simulink model "one"  (R2021a)
settings: Solver=ode45  StartTime=0.0  StopTime=50.0  MaxStep=0.05  RelTol=1e-3
libraries: pid_lib x1
settings Model: Creator=jeffr  LastModifiedBy=jeffr

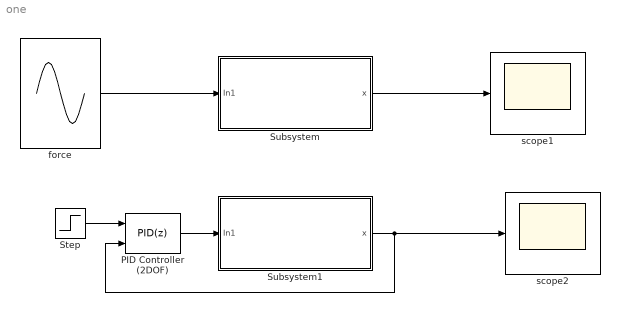
== system one ==
  PID Controller (2DOF) : pid_lib/PID Controller (2DOF)  Controller=PID  Form=Parallel  TimeDomain=Discrete-time  UseExternalTs=off  SampleTime=0.01  IntegratorMethod=Forward Euler  FilterMethod=Forward Euler  ControllerParametersSource=internal  P=1  I=1  D=0  UseFilter=on  N=100  b=1  c=1  TunerSelectOption=Transfer Function Based (PID Tuner App)  InitialConditionSource=internal  InitialConditionForIntegrator=0  InitialConditionForFilter=0  DifferentiatorICPrevScaledInput=0  ExternalReset=none  TrackingMode=off  Kt=1  LimitOutput=off  SatLimitsSource=internal  UpperSaturationLimit=inf  LowerSaturationLimit=-inf  LinearizeAsGain=on  AntiWindupMode=none  Kb=1  POutMin=[]  POutMax=[]  IOutMin=[]  IOutMax=[]  DOutMin=[]  DOutMax=[]  NOutMin=[]  NOutMax=[]  bOutMin=[]  bOutMax=[]  cOutMin=[]  cOutMax=[]  SumOutMin=[]  SumOutMax=[]  SaturationOutMin=[]  SaturationOutMax=[]  PParamMin=[]  PParamMax=[]  IParamMin=[]  IParamMax=[]  DParamMin=[]  DParamMax=[]  NParamMin=[]  NParamMax=[]  bParamMin=[]  bParamMax=[]  cParamMin=[]  cParamMax=[]  KbParamMin=[]  KbParamMax=[]  KtParamMin=[]  KtParamMax=[]  KbOutMin=[]  KbOutMax=[]  KtOutMin=[]  KtOutMax=[]  IntegratorOutMin=[]  IntegratorOutMax=[]  FilterOutMin=[]  FilterOutMax=[]  SumI1OutMin=[]  SumI1OutMax=[]  SumI2OutMin=[]  SumI2OutMax=[]  SumI3OutMin=[]  SumI3OutMax=[]  SumI4OutMin=[]  SumI4OutMax=[]  SumDOutMin=[]  SumDOutMax=[]  Sum1OutMin=[]  Sum1OutMax=[]  Sum2OutMin=[]  Sum2OutMax=[]  Sum3OutMin=[]  Sum3OutMax=[]  DifferentiatorOutMin=[]  DifferentiatorOutMax=[]  FilterDiffOutCoefMin=[]  FilterDiffOutCoefMax=[]  ReciprocalOutMin=[]  ReciprocalOutMax=[]  SumDenOutMin=[]  SumDenOutMax=[]  SumNumOutMin=[]  SumNumOutMax=[]  DivideOutMin=[]  DivideOutMax=[]  UdiffTsProdOutMin=[]  UdiffTsProdOutMax=[]  NTsProdOutMin=[]  NTsProdOutMax=[]  UintegralTsProdOutMin=[]  UintegralTsProdOutMax=[]  UngainTsProdOutMin=[]  UngainTsProdOutMax=[]  IntegratorContinuousStateAttributes=''  IntegratorStateMustResolveToSignalObject=off  IntegratorRTWStateStorageClass=Auto  FilterContinuousStateAttributes=''  FilterStateMustResolveToSignalObject=off  FilterRTWStateStorageClass=Auto  ParallelPVariant=InternalParameters  IdealPVariant=Disabled  IVariant=InternalParameters  DVariant=InternalParameters  bVariant=InternalParameters  cVariant=InternalParameters  IntegratorVariant=Discrete  SatVariant=Disabled  AWVariant=Passthrough  PCopyVariant=Disabled  TRVariant=Disabled  FdbkBlocksVariant=Forward  IdealPFdbkVariant=Disabled  SatFdbkVariant=Disabled  DerivativeFilterVariant=ForwardEulerFilter  NVariant=InternalParameters  NCopyVariant=Disabled  FilterICVariant=InternalICsFilter  IntegratorICVariant=InternalICs  ExternalResetVariant=Disabled  TRSumVariant=Passthrough  SumFdbkVariant=Disabled  SumVariant=Sum_PID  TsampFilterVariant=InternalTs  TsampNgainVariant=Passthrough  TsampIntegralVariant=Passthrough  ExternalSaturationOutDataTypeStr=Inherit: Same as second input
      settings: SourceProductBaseCode=SL
  Step : Step  SampleTime=0
  Subsystem : Subsystem  mask{m=1, k=0.2, b=0.1}
      mask prompts: m "mass"; k "spring"; b "damper"
      mask Display: disp('my subsystem')
  Subsystem1 : Subsystem  mask{m=1, k=0.2, b=0.1}
      mask prompts: m "mass"; k "spring"; b "damper"
      mask Display: disp('my subsystem')
  force : Sin  Amplitude=2  SampleTime=0
  scope1 : Scope
  scope2 : Scope
  wires:
  force/1 -> Subsystem/1(In1)
  Subsystem/1(x) -> scope1/1
  PID Controller (2DOF)/1 -> Subsystem1/1(In1)
  Subsystem1/1(x) -> PID Controller (2DOF)/2, scope2/1
  Step/1 -> PID Controller (2DOF)/1

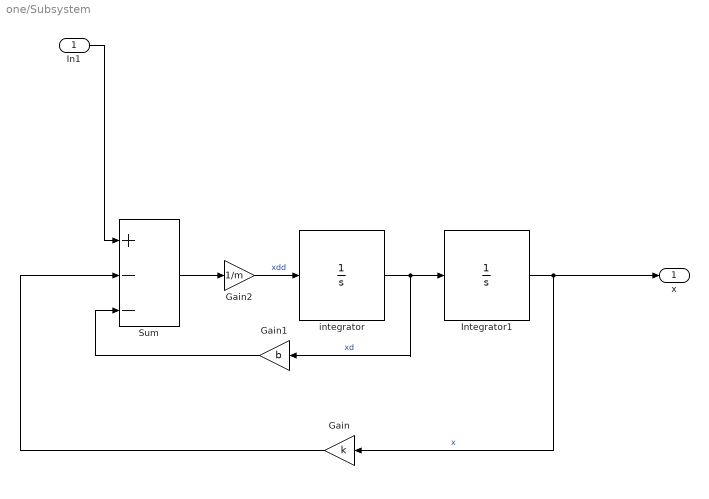
== system one/Subsystem ==
  In1 : Inport
  Gain : Gain  Gain=k
  Gain1 : Gain  Gain=b
  Gain2 : Gain  Gain=1/m
  Integrator1 : Integrator
  Sum : Sum  Inputs=|+--
  integrator : Integrator
  x : Outport
  wires:
  Integrator1/1 -> x/1, Gain/1  "x"
  integrator/1 -> Gain1/1, Integrator1/1  "xd"
  In1/1 -> Sum/1
  Gain2/1 -> integrator/1  "xdd"
  Gain1/1 -> Sum/3
  Gain/1 -> Sum/2
  Sum/1 -> Gain2/1

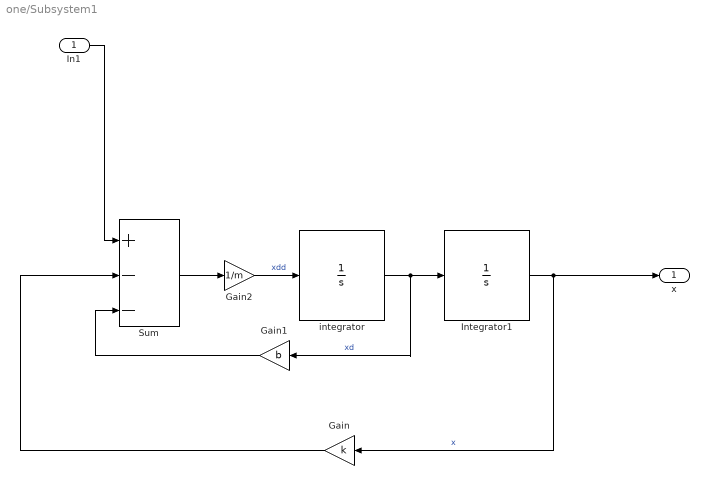
== system one/Subsystem1 ==
  In1 : Inport
  Gain : Gain  Gain=k
  Gain1 : Gain  Gain=b
  Gain2 : Gain  Gain=1/m
  Integrator1 : Integrator
  Sum : Sum  Inputs=|+--
  integrator : Integrator
  x : Outport
  wires:
  Sum/1 -> Gain2/1
  Gain/1 -> Sum/2
  Gain1/1 -> Sum/3
  Gain2/1 -> integrator/1  "xdd"
  In1/1 -> Sum/1
  integrator/1 -> Integrator1/1, Gain1/1  "xd"
  Integrator1/1 -> Gain/1, x/1  "x"
